simulink model "red6Rossler_corregido"  (Simulink 7.9)
settings: Solver=ode23tb  StartTime=0.0  StopTime=30  RelTol=1e-3
values from neighbouring files (symbols this model uses):
  a = 0.1    [param_Ross.m]
  amp = .2    (= 0.2)    [param_Ross.m]
  b = 4    [param_Ross.m]
  d = 2    [param_Ross.m]
  K = 1    [param_Ross.m]
  ofs = 1    [param_Ross.m]
settings Model: Creator=zapata131  LastModifiedBy=zapata131
settings GRTTargetCC: CombineOutputUpdateFcns=off  GRTInterface=on

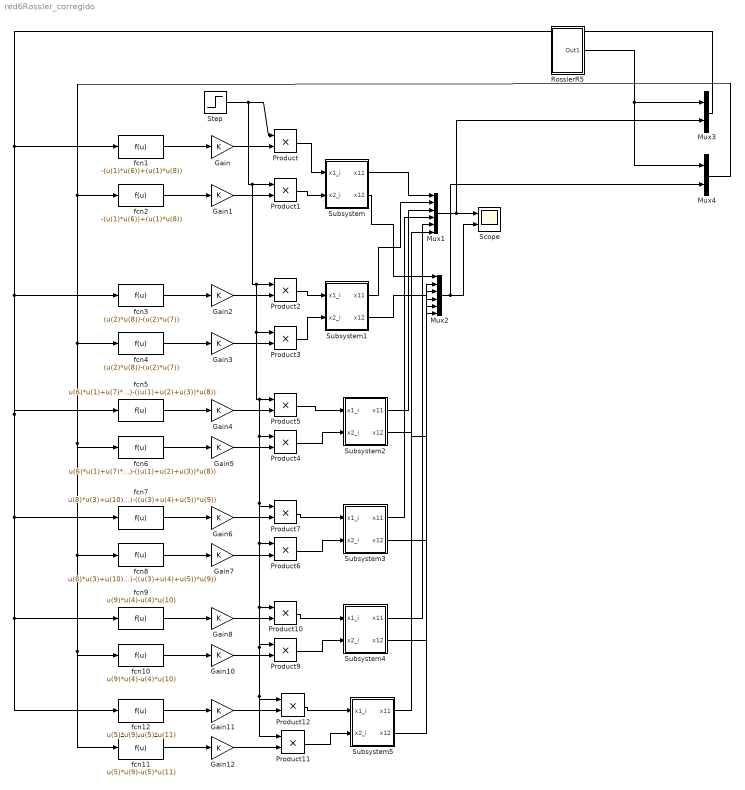
== system red6Rossler_corregido ==
  Gain{,1..8,10..12} (12 alike) : Gain  Gain=K
  Mux1 : Mux  Inputs=6
  Mux2 : Mux  Inputs=6
  Mux3 : Mux  Inputs=2
  Mux4 : Mux  Inputs=2
  Product{,1..7,9..12} (12 alike) : Product  RndMeth=Zero
  RosslerR5 : Subsystem
  Scope : Scope  NumInputPorts=2
      settings: TickLabels=on  TimeRange=12  YMin=-25~-40  YMax=15~30
  Step : Step  Time=15  SampleTime=0
  Subsystem : Subsystem
  Subsystem1 : Subsystem
  Subsystem2 : Subsystem
  Subsystem3 : Subsystem
  Subsystem4 : Subsystem
  Subsystem5 : Subsystem
  fcn1 : Fcn  Expr=-(u(1)*u(6))+(u(1)*u(8))
  fcn10 : Fcn  Expr=u(9)*u(4)-u(4)*u(10)
  fcn11 : Fcn  Expr=u(5)*u(9)-u(5)*u(11)
  fcn12 : Fcn  Expr=u(5)*u(9)-u(5)*u(11)
  fcn2 : Fcn  Expr=-(u(1)*u(6))+(u(1)*u(8))
  fcn3 : Fcn  Expr=(u(2)*u(8))-(u(2)*u(7))
  fcn4 : Fcn  Expr=(u(2)*u(8))-(u(2)*u(7))
  fcn5 : Fcn  Expr=u(6)*u(1)+u(7)*u(2)+u(9)*u(3)-((u(1)+u(2)+u(3))*u(8))
  fcn6 : Fcn  Expr=u(6)*u(1)+u(7)*u(2)+u(9)*u(3)-((u(1)+u(2)+u(3))*u(8))
  fcn7 : Fcn  Expr=u(8)*u(3)+u(10)*u(4)+u(11)*u(5)-((u(3)+u(4)+u(5))*u(9))
  fcn8 : Fcn  Expr=u(8)*u(3)+u(10)*u(4)+u(11)*u(5)-((u(3)+u(4)+u(5))*u(9))
  fcn9 : Fcn  Expr=u(9)*u(4)-u(4)*u(10)
  wires:
  Subsystem/1(x11) -> Mux1/1
  Subsystem1/1(x11) -> Mux1/2
  Subsystem2/1(x11) -> Mux1/3
  Subsystem/2(x12) -> Mux2/1
  Subsystem1/2(x12) -> Mux2/2
  Subsystem2/2(x12) -> Mux2/3
  Mux1/1 -> Mux3/2, Scope/1
  Product/1 -> Subsystem/1(x1_i)
  Step/1 -> Product/1, Product1/1, Product2/1, Product3/1, Product5/1, Product4/1, Product7/1, Product6/1, Product10/1, Product9/1, Product12/1, Product11/1
  Product1/1 -> Subsystem/2(x2_i)
  Product3/1 -> Subsystem1/2(x2_i)
  Product2/1 -> Subsystem1/1(x1_i)
  Product4/1 -> Subsystem2/2(x2_i)
  Product5/1 -> Subsystem2/1(x1_i)
  Gain/1 -> Product/2
  Gain1/1 -> Product1/2
  Gain2/1 -> Product2/2
  Gain3/1 -> Product3/2
  Gain4/1 -> Product5/2
  Gain5/1 -> Product4/2
  Mux2/1 -> Scope/2, Mux4/2
  Product6/1 -> Subsystem3/2(x2_i)
  Product7/1 -> Subsystem3/1(x1_i)
  Gain6/1 -> Product7/2
  Gain7/1 -> Product6/2
  Product9/1 -> Subsystem4/2(x2_i)
  Product10/1 -> Subsystem4/1(x1_i)
  Gain8/1 -> Product10/2
  Gain10/1 -> Product9/2
  Product11/1 -> Subsystem5/2(x2_i)
  Product12/1 -> Subsystem5/1(x1_i)
  Gain11/1 -> Product12/2
  Gain12/1 -> Product11/2
  Subsystem3/1(x11) -> Mux1/4
  Subsystem3/2(x12) -> Mux2/4
  Subsystem4/1(x11) -> Mux1/5
  Subsystem4/2(x12) -> Mux2/5
  Subsystem5/1(x11) -> Mux1/6
  Subsystem5/2(x12) -> Mux2/6
  RosslerR5/1(Out1) -> Mux3/1, Mux4/1
  fcn1/1 -> Gain/1
  fcn2/1 -> Gain1/1
  fcn3/1 -> Gain2/1
  fcn4/1 -> Gain3/1
  fcn5/1 -> Gain4/1
  fcn6/1 -> Gain5/1
  fcn7/1 -> Gain6/1
  fcn8/1 -> Gain7/1
  fcn9/1 -> Gain8/1
  fcn10/1 -> Gain10/1
  fcn12/1 -> Gain11/1
  fcn11/1 -> Gain12/1
  Mux4/1 -> fcn11/1, fcn10/1, fcn8/1, fcn6/1, fcn4/1, fcn2/1
  Mux3/1 -> fcn3/1, fcn5/1, fcn7/1, fcn12/1, fcn9/1, fcn1/1

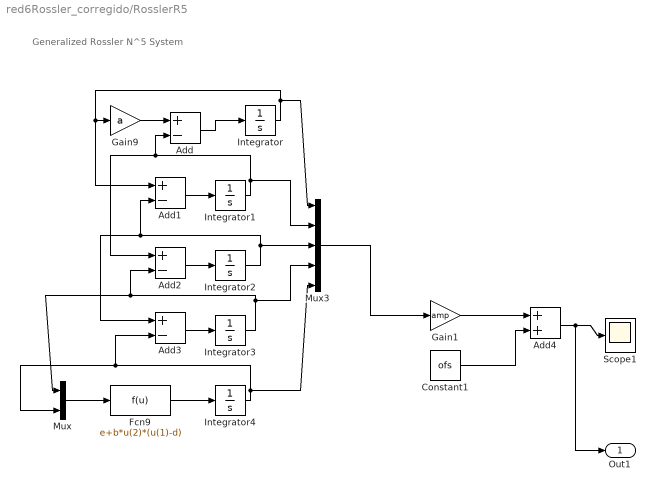
== system red6Rossler_corregido/RosslerR5 ==
  note: Generalized Rossler N^5 System
  Add{,1..3} (4 alike) : Sum  Inputs=+-
  Add4 : Sum
  Constant1 : Constant  Value=ofs
  Fcn9 : Fcn  Expr=e+b*u(2)*(u(1)-d)
  Gain1 : Gain  Gain=amp
  Gain9 : Gain  Gain=a
  Integrator : Integrator  InitialCondition=0.1
  Integrator1 : Integrator
  Integrator2 : Integrator  InitialCondition=-1
  Integrator3 : Integrator
  Integrator4 : Integrator  InitialCondition=1
  Mux : Mux  Inputs=2
  Mux3 : Mux  Inputs=5
  Scope1 : Scope
  Out1 : Outport
  wires:
  Integrator/1 -> Gain9/1, Add1/1, Mux3/1
  Gain9/1 -> Add/1
  Add/1 -> Integrator/1
  Integrator1/1 -> Add/2, Add2/1, Mux3/2
  Add1/1 -> Integrator1/1
  Integrator2/1 -> Add1/2, Add3/1, Mux3/3
  Add2/1 -> Integrator2/1
  Integrator3/1 -> Add2/2, Mux/1, Mux3/4
  Add3/1 -> Integrator3/1
  Integrator4/1 -> Add3/2, Mux/2, Mux3/5
  Fcn9/1 -> Integrator4/1
  Mux/1 -> Fcn9/1
  Constant1/1 -> Add4/2
  Gain1/1 -> Add4/1
  Add4/1 -> Scope1/1, Out1/1
  Mux3/1 -> Gain1/1

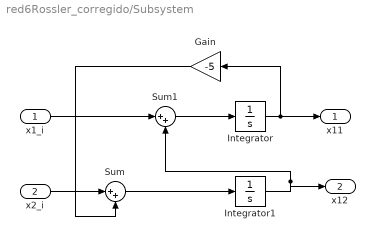
== system red6Rossler_corregido/Subsystem ==
  x1_i : Inport
  x2_i : Inport  Port=2
  Gain : Gain  Gain=-5
  Integrator : Integrator  InitialCondition=10
  Integrator1 : Integrator  InitialCondition=1
  Sum : Sum  Inputs=|++
  Sum1 : Sum  Inputs=|++
  x11 : Outport
  x12 : Outport  Port=2
  wires:
  x2_i/1 -> Sum/1
  Integrator/1 -> Gain/1, x11/1
  Gain/1 -> Sum/2
  Sum/1 -> Integrator1/1
  Integrator1/1 -> Sum1/2, x12/1
  x1_i/1 -> Sum1/1
  Sum1/1 -> Integrator/1

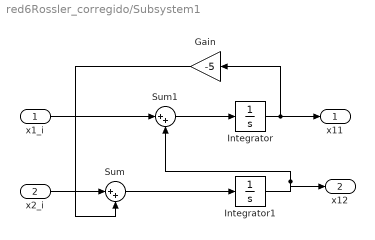
== system red6Rossler_corregido/Subsystem1 ==
  x1_i : Inport
  x2_i : Inport  Port=2
  Gain : Gain  Gain=-5
  Integrator : Integrator  InitialCondition=-10
  Integrator1 : Integrator  InitialCondition=2
  Sum : Sum  Inputs=|++
  Sum1 : Sum  Inputs=|++
  x11 : Outport
  x12 : Outport  Port=2
  wires:
  x2_i/1 -> Sum/1
  Integrator/1 -> Gain/1, x11/1
  Gain/1 -> Sum/2
  Sum/1 -> Integrator1/1
  Integrator1/1 -> Sum1/2, x12/1
  x1_i/1 -> Sum1/1
  Sum1/1 -> Integrator/1

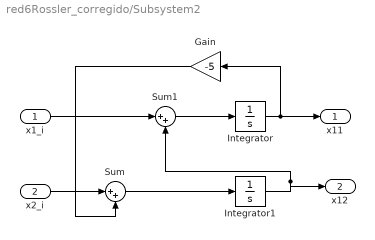
== system red6Rossler_corregido/Subsystem2 ==
  x1_i : Inport
  x2_i : Inport  Port=2
  Gain : Gain  Gain=-5
  Integrator : Integrator  InitialCondition=-8
  Integrator1 : Integrator  InitialCondition=10
  Sum : Sum  Inputs=|++
  Sum1 : Sum  Inputs=|++
  x11 : Outport
  x12 : Outport  Port=2
  wires:
  x2_i/1 -> Sum/1
  Integrator/1 -> Gain/1, x11/1
  Gain/1 -> Sum/2
  Sum/1 -> Integrator1/1
  Integrator1/1 -> Sum1/2, x12/1
  x1_i/1 -> Sum1/1
  Sum1/1 -> Integrator/1

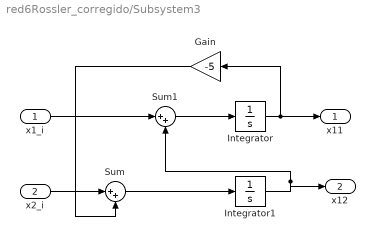
== system red6Rossler_corregido/Subsystem3 ==
  x1_i : Inport
  x2_i : Inport  Port=2
  Gain : Gain  Gain=-5
  Integrator : Integrator  InitialCondition=-3
  Integrator1 : Integrator  InitialCondition=10
  Sum : Sum  Inputs=|++
  Sum1 : Sum  Inputs=|++
  x11 : Outport
  x12 : Outport  Port=2
  wires:
  x2_i/1 -> Sum/1
  Integrator/1 -> Gain/1, x11/1
  Gain/1 -> Sum/2
  Sum/1 -> Integrator1/1
  Integrator1/1 -> Sum1/2, x12/1
  x1_i/1 -> Sum1/1
  Sum1/1 -> Integrator/1

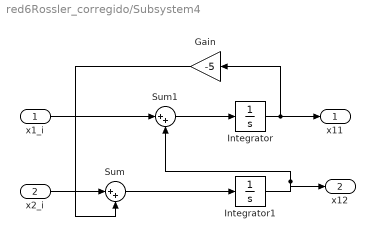
== system red6Rossler_corregido/Subsystem4 ==
  x1_i : Inport
  x2_i : Inport  Port=2
  Gain : Gain  Gain=-5
  Integrator : Integrator  InitialCondition=-9
  Integrator1 : Integrator  InitialCondition=8
  Sum : Sum  Inputs=|++
  Sum1 : Sum  Inputs=|++
  x11 : Outport
  x12 : Outport  Port=2
  wires:
  x2_i/1 -> Sum/1
  Integrator/1 -> Gain/1, x11/1
  Gain/1 -> Sum/2
  Sum/1 -> Integrator1/1
  Integrator1/1 -> Sum1/2, x12/1
  x1_i/1 -> Sum1/1
  Sum1/1 -> Integrator/1

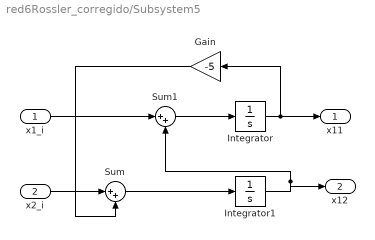
== system red6Rossler_corregido/Subsystem5 ==
  x1_i : Inport
  x2_i : Inport  Port=2
  Gain : Gain  Gain=-5
  Integrator : Integrator  InitialCondition=-5
  Integrator1 : Integrator  InitialCondition=11
  Sum : Sum  Inputs=|++
  Sum1 : Sum  Inputs=|++
  x11 : Outport
  x12 : Outport  Port=2
  wires:
  x2_i/1 -> Sum/1
  Integrator/1 -> Gain/1, x11/1
  Gain/1 -> Sum/2
  Sum/1 -> Integrator1/1
  Integrator1/1 -> Sum1/2, x12/1
  x1_i/1 -> Sum1/1
  Sum1/1 -> Integrator/1
